simulink model "sim_topic1"  (R2023a)
settings: Solver=VariableStepAuto  StartTime=0.0  StopTime=N  RelTol=1e-3
settings Model: Creator=user  LastModifiedBy=user

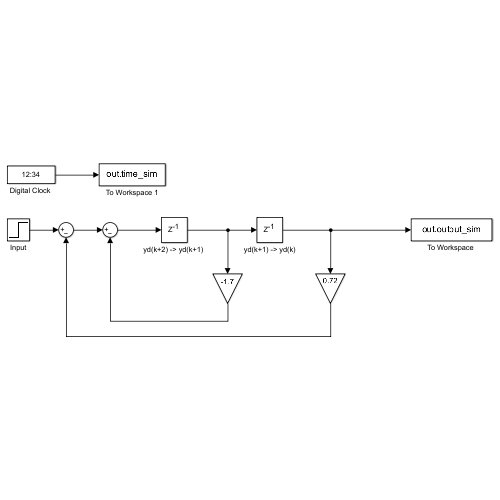
[thumbnail: Simulink's stored preview of the top-level diagram]
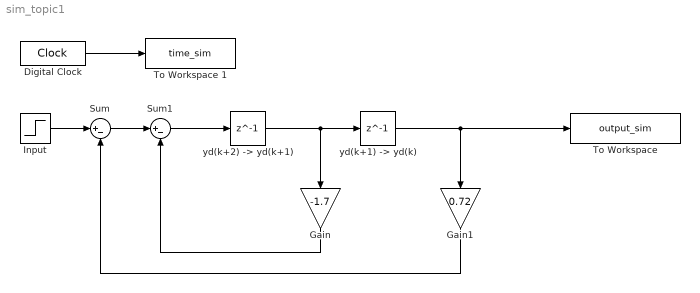
== system sim_topic1 ==
  "Digital Clock " : DigitalClock
  Gain : Gain  Gain=-1.7
  Gain1 : Gain  Gain=0.72
  Input : Step  Time=0  SampleTime=1
  Sum : Sum  Inputs=|+-
  Sum1 : Sum  Inputs=|+-
  "To Workspace " : ToWorkspace  VariableName=output_sim  SampleTime=-1
  To Workspace 1 : ToWorkspace  VariableName=time_sim  SampleTime=-1
  "yd(k+1) -> yd(k)" : Delay  DelayLength=1  InitialCondition=1
  "yd(k+2) -> yd(k+1) " : Delay  DelayLength=1  InitialCondition=2
  wires:
  "yd(k+2) -> yd(k+1) "/1 -> Gain/1, "yd(k+1) -> yd(k)"/1
  Input/1 -> Sum/1
  "yd(k+1) -> yd(k)"/1 -> "To Workspace "/1, Gain1/1
  Gain/1 -> Sum1/2
  Sum/1 -> Sum1/1
  Sum1/1 -> "yd(k+2) -> yd(k+1) "/1
  Gain1/1 -> Sum/2
  "Digital Clock "/1 -> To Workspace 1/1
